simulink model "week3_que4"  (R2020b)
settings: Solver=ode15s  StartTime=0.0  StopTime=0.002  RelTol=1e-3
model workspace (MAT data in the model file):
  J = 3.2284e-06
  K = 0.0274
  L = 2.75e-06
  R = 4
  b = 3.5077e-06
  k = 0.0274
settings Model: Creator=mluser  LastModifiedBy=mluser

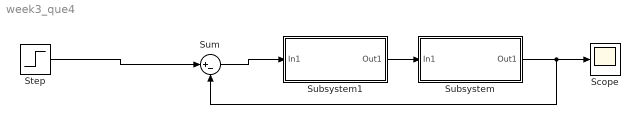
== system week3_que4 ==
  Scope : Scope
  Step : Step  Time=0  SampleTime=0
  Subsystem : Subsystem
  Subsystem1 : Subsystem
  Sum : Sum  Inputs=|+-
  wires:
  Subsystem/1(Out1) -> Sum/2, Scope/1
  Sum/1 -> Subsystem1/1(In1)
  Subsystem1/1(Out1) -> Subsystem/1(In1)
  Step/1 -> Sum/1

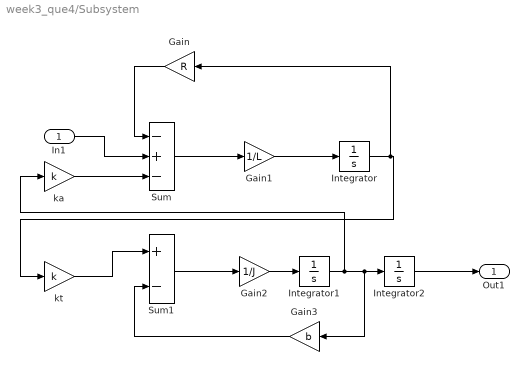
== system week3_que4/Subsystem ==
  In1 : Inport
  Gain : Gain  Gain=R
  Gain1 : Gain  Gain=1/L
  Gain2 : Gain  Gain=1/J
  Gain3 : Gain  Gain=b
  Integrator : Integrator
  Integrator1 : Integrator
  Integrator2 : Integrator
  Sum : Sum  Inputs=-+-
  Sum1 : Sum  Inputs=+-
  ka : Gain  Gain=k
  kt : Gain  Gain=k
  Out1 : Outport
  wires:
  Integrator/1 -> Gain/1, kt/1
  Gain3/1 -> Sum1/2
  Gain2/1 -> Integrator1/1
  Gain1/1 -> Integrator/1
  ka/1 -> Sum/3
  Integrator1/1 -> ka/1, Gain3/1, Integrator2/1
  Sum/1 -> Gain1/1
  Sum1/1 -> Gain2/1
  kt/1 -> Sum1/1
  Gain/1 -> Sum/1
  Integrator2/1 -> Out1/1
  In1/1 -> Sum/2

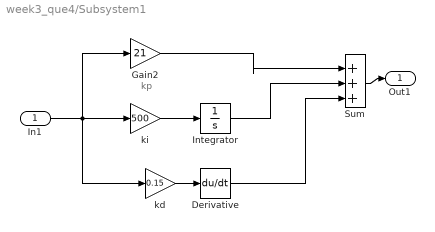
== system week3_que4/Subsystem1 ==
  note: kp
  In1 : Inport
  Derivative : Derivative
  Gain2 : Gain  Gain=21
  Integrator : Integrator
  Sum : Sum  Inputs=|+++
  kd : Gain  Gain=0.15
  ki : Gain  Gain=500
  Out1 : Outport
  wires:
  kd/1 -> Derivative/1
  In1/1 -> kd/1, Gain2/1, ki/1
  Gain2/1 -> Sum/1
  ki/1 -> Integrator/1
  Integrator/1 -> Sum/2
  Derivative/1 -> Sum/3
  Sum/1 -> Out1/1
